simulink model "Ycap_snt"  (R2025b)
settings: Solver=ode45  StartTime=0.0  StopTime=10.0  RelTol=1e-3  EnableMultiTasking=on
undefined symbols (not defined in the file or in its folder): DiscIntNeverNeededParam, Ts
libraries: fl_lib x24, nesl_utility x12
(part 1 of 3)
settings Model: Creator=gdudgeon  LastModifiedBy=gdudgeon
settings SolverCC: AlgebraicLoopSolver=TrustRegion
settings DataIOCC: LimitDataPoints=on  SaveFormat=Array  ReturnWorkspaceOutputs=off
settings OptimizationCC: LifeSpan=inf
settings DebuggingCC: UnderspecifiedInitializationDetection=Classic  MergeDetectMultiDrivingBlocksExec=none  SolverPrmCheckMsg=warning  UnconnectedInputMsg=warning  UnconnectedOutputMsg=warning  UnconnectedLineMsg=warning  StateNameClashWarn=warning  SFUnexpectedBacktrackingDiag=warning  SFNoUnconditionalDefaultTransitionDiag=warning  SFExecutionAtInitializationDiag=none  ArithmeticOperatorsInVariantConditions=warning
settings HardwareCC: ProdBitPerPointer=32.0  ProdBitPerSizeT=32.0  ProdBitPerPtrDiffT=32.0  ProdLargestAtomicFloat=None  ProdIntDivRoundTo=Undefined  ProdEndianess=Unspecified  ProdWordSize=32.0  ProdHWDeviceType=32-bit Generic
settings ModelReferenceCC: EnableRefExpFcnMdlSchedulingChecks=on  PropagateSignalLabelsOutOfModel=off
settings SFSimCC: SimUseLocalCustomCode=off  CustomCodeUndefinedFunction=UseInterfaceOnly
settings RTWCC: RTWUseLocalCustomCode=off  GPUComputeCapability=3.5
settings CodeAppCC: StateflowObjectComments=on
settings GRTTargetCC: TargetLangStandard=C89/C90 (ANSI)
settings ConfigComp: CovMetricSettings=dw  CovSaveCumulativeToWorkspaceVar=on  CovSaveSingleToWorkspaceVar=on  CovExternalEMLEnable=off
settings SimscapeCC: SimscapeNormalizeSystem=off

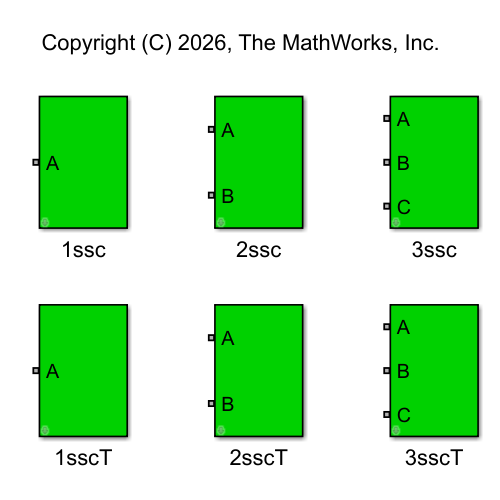
[thumbnail: Simulink's stored preview of the top-level diagram]
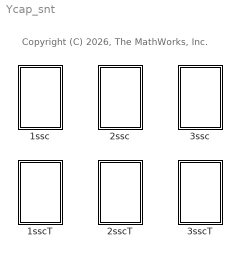
== system Ycap_snt ==
  note: Copyright (C) 2026, The MathWorks, Inc.
  1ssc : Subsystem  mask{V=4.16e3, Qc=50e3}
      mask prompts: V "Vrms (V)"; Qc "Reactive power (VAr)"
  1sscT : Subsystem  mask{V=4.16e3, Qc=50e3}
      mask prompts: V "Vrms (V)"; Qc "Reactive power (VAr)"
  2ssc : Subsystem  mask{V=4.16e3, Qc=50e3}
      mask prompts: V "Vrms (V)"; Qc "Reactive power (VAr)"
  2sscT : Subsystem  mask{V=4.16e3, Qc=50e3}
      mask prompts: V "Vrms (V)"; Qc "Reactive power (VAr)"
  3ssc : Subsystem  mask{V=4.16e3, Qc=200e3}
      mask prompts: V "Vrms (V)"; Qc "Reactive power (VAr)"
  3sscT : Subsystem  mask{V=4.16e3, Qc=200e3}
      mask prompts: V "Vrms (V)"; Qc "Reactive power (VAr)"

== system Ycap_snt/1ssc ==
  Electrical Reference : fl_lib/Electrical/Electrical Elements/Electrical Reference
  cap load : Subsystem  mask{Vrms=V/sqrt(3), f=60, P=0, Q=Qc}
      mask prompts: Vrms "Vrms (V)"; f "freq (Hz)"; P "P (W)"; Q "Q (VA)"
      mask init:
      | R = Vrms^2*P/(P^2 + Q^2);
      | 
      | C = (P^2 + Q^2)/(2*pi*f)/Vrms^2/Q;
  A : PMIOPort  Side=Left
  connections:
  Electrical Reference/LConn1 -- cap load/RConn1
  A/RConn1 -- cap load/LConn1

== system Ycap_snt/1sscT ==
  Constant : Constant  Value=[0 -Qc]  SampleTime=-1
  Electrical Reference1 : fl_lib/Electrical/Electrical Elements/Electrical Reference
  constPQ1 : Subsystem
  A : PMIOPort  Side=Left
  wires:
  Constant/1 -> constPQ1/1(PQ)
  connections:
  constPQ1/RConn1 -- A/RConn1
  constPQ1/LConn1 -- Electrical Reference1/LConn1

== system Ycap_snt/2ssc ==
  Electrical Reference : fl_lib/Electrical/Electrical Elements/Electrical Reference
  cap load : Subsystem  mask{Vrms=V/sqrt(3), f=60, P=0, Q=Qc}
      mask prompts: Vrms "Vrms (V)"; f "freq (Hz)"; P "P (W)"; Q "Q (VA)"
      mask init:
      | R = Vrms^2*P/(P^2 + Q^2);
      | 
      | C = (P^2 + Q^2)/(2*pi*f)/Vrms^2/Q;
  cap load1 : Subsystem  mask{Vrms=V/sqrt(3), f=60, P=0, Q=Qc}
      mask prompts: Vrms "Vrms (V)"; f "freq (Hz)"; P "P (W)"; Q "Q (VA)"
      mask init:
      | R = Vrms^2*P/(P^2 + Q^2);
      | 
      | C = (P^2 + Q^2)/(2*pi*f)/Vrms^2/Q;
  A : PMIOPort  Side=Left
  B : PMIOPort  Port=2  Side=Left
  connections:
  cap load1/LConn1 -- B/RConn1
  cap load/LConn1 -- A/RConn1
  Electrical Reference/LConn1 -- cap load1/RConn1 -- cap load/RConn1

== system Ycap_snt/2sscT ==
  Constant : Constant  Value=[0 -Qc]  SampleTime=-1
  Electrical Reference : fl_lib/Electrical/Electrical Elements/Electrical Reference
  constPQ1 : Subsystem
  constPQ2 : Subsystem
  A : PMIOPort  Side=Left
  B : PMIOPort  Port=2  Side=Left
  wires:
  Constant/1 -> constPQ2/1(PQ), constPQ1/1(PQ)
  connections:
  constPQ1/RConn1 -- A/RConn1
  constPQ2/RConn1 -- B/RConn1
  Electrical Reference/LConn1 -- constPQ2/LConn1 -- constPQ1/LConn1

== system Ycap_snt/3ssc ==
  Electrical Reference : fl_lib/Electrical/Electrical Elements/Electrical Reference
  cap load : Subsystem  mask{Vrms=V/sqrt(3), f=60, P=0, Q=Qc}
      mask prompts: Vrms "Vrms (V)"; f "freq (Hz)"; P "P (W)"; Q "Q (VA)"
      mask init:
      | R = Vrms^2*P/(P^2 + Q^2);
      | 
      | C = (P^2 + Q^2)/(2*pi*f)/Vrms^2/Q;
  cap load1 : Subsystem  mask{Vrms=V/sqrt(3), f=60, P=0, Q=Qc}
      mask prompts: Vrms "Vrms (V)"; f "freq (Hz)"; P "P (W)"; Q "Q (VA)"
      mask init:
      | R = Vrms^2*P/(P^2 + Q^2);
      | 
      | C = (P^2 + Q^2)/(2*pi*f)/Vrms^2/Q;
  cap load2 : Subsystem  mask{Vrms=V/sqrt(3), f=60, P=0, Q=Qc}
      mask prompts: Vrms "Vrms (V)"; f "freq (Hz)"; P "P (W)"; Q "Q (VA)"
      mask init:
      | R = Vrms^2*P/(P^2 + Q^2);
      | 
      | C = (P^2 + Q^2)/(2*pi*f)/Vrms^2/Q;
  A : PMIOPort  Side=Left
  B : PMIOPort  Port=2  Side=Left
  C : PMIOPort  Port=3  Side=Left
  connections:
  cap load2/LConn1 -- C/RConn1
  cap load1/LConn1 -- B/RConn1
  cap load/LConn1 -- A/RConn1
  Electrical Reference/LConn1 -- cap load2/RConn1 -- cap load1/RConn1 -- cap load/RConn1

== system Ycap_snt/3sscT ==
  Constant : Constant  Value=[0 -Qc]  SampleTime=-1
  Electrical Reference : fl_lib/Electrical/Electrical Elements/Electrical Reference
  constPQ1 : Subsystem
  constPQ2 : Subsystem
  constPQ3 : Subsystem
  A : PMIOPort  Side=Left
  B : PMIOPort  Port=2  Side=Left
  C : PMIOPort  Port=3  Side=Left
  wires:
  Constant/1 -> constPQ3/1(PQ), constPQ2/1(PQ), constPQ1/1(PQ)
  connections:
  constPQ1/RConn1 -- A/RConn1
  constPQ2/RConn1 -- B/RConn1
  constPQ3/RConn1 -- C/RConn1
  Electrical Reference/LConn1 -- constPQ3/LConn1 -- constPQ2/LConn1 -- constPQ1/LConn1

== system Ycap_snt/1ssc/cap load ==
  Capacitor : fl_lib/Electrical/Electrical Elements/Capacitor  c=C F  r=R Ohm  g=0 1/Ohm  i_specify=on  i_priority=Low  i=0 A  i_nominal_specify=off  i_nominal_value=1  i_nominal_unit=A  v_specify=on  v_priority=Low  v=0 V  v_nominal_specify=off  v_nominal_value=1  v_nominal_unit=V  vc_specify=on  vc_priority=Low  vc=0 V  vc_nominal_specify=off  vc_nominal_value=1  vc_nominal_unit=V
  " +" : PMIOPort  Side=Left
  - : PMIOPort  Port=2  Side=Right
  connections:
  Capacitor/LConn1 -- " +"/RConn1
  Capacitor/RConn1 -- -/RConn1

== system Ycap_snt/1sscT/constPQ1 ==
  PQ : Inport
  Controlled Current Source : fl_lib/Electrical/Electrical Sources/Controlled Current Source
  Demux : Demux  Outputs=2
  PS-Simulink Converter : nesl_utility/PS-Simulink Converter  PhysicalDomain=network_engine_domain  SubClassName=ps_output  LeftPortType=input  RightPortType=output  PseudoPeriodic=off  Frequencies=[]  VectorFormat=inherit  Unit=inherit  AffineConversion=off
  Simulink-PS Converter : nesl_utility/Simulink-PS Converter  PhysicalDomain=network_engine_domain  SubClassName=ps_input  LeftPortType=input  RightPortType=output  PseudoPeriodic=off  Frequencies=[]  NoiseDistribution=none  NoiseParameters=[]  Unit=1  AffineConversion=off  FilteringAndDerivatives=zero  SimscapeFilterOrder=1  InputFilterTimeConstant=0.001  UdotUserProvided=0
  Voltage Sensor : fl_lib/Electrical/Electrical Sensors/Voltage Sensor
  single-phase PQ : Subsystem
      settings: PortSchema="{\"entries\":[{\"content\":{\"sides\":[{\"content\":{\"connectorIds\":[\"In1\",\"In2\"]},\"type\":\"ConnectorPlacement.EquallySpacedRectSide\",\"uuid\":\"dcb77ad6-d65a-4afe-9b75-44cea2e03bc8\"},{\"content\":{\"connectorIds\":[\"Out1\"],\"side\":\"RIGHT\"},\"type\":\"ConnectorPlacement.EquallySpacedRectSide\",\"uuid\":\"20550ec8-912f-4e6b-8efc-55d7f6680ac4\"},{\"content\":{\"side\":\"TOP\"},\"type\":\"ConnectorPlacement.EquallySpacedRectSide\",\"uuid\":\"6ad8cbf4-1495-4620-97d9-4b8af34d00d1\"},{\"content\":{\"connectorIds\":[\"In3\"],\"side\":\"BOTTOM\"},\"type\":\"ConnectorPlacement.EquallySpacedRectSide\",\"uuid\":\"0b9a8788-8400-4a69-9d07-dd0028530e33\"}]},\"type\":\"ConnectorPlacement.EquallySpacedConnector\",\"uuid\":\"b57ec49b-aa32-43b3-a026-14ed90072d63\"}],\"packageUris\":[\"http://schema.mathworks.com/mf0/Connector/R2020b\"],\"version\":\"1.0\"}"
  + : PMIOPort  Side=Right
  - : PMIOPort  Port=2  Side=Left
  wires:
  PS-Simulink Converter/1 -> single-phase PQ/3(meas)
  single-phase PQ/1(I_1ph) -> Simulink-PS Converter/1
  Demux/1 -> single-phase PQ/1(P)
  Demux/2 -> single-phase PQ/2(Q)
  PQ/1 -> Demux/1
  connections:
  Controlled Current Source/RConn2 -- -/RConn1 -- Voltage Sensor/RConn2
  Voltage Sensor/LConn1 -- +/RConn1 -- Controlled Current Source/LConn1
  PS-Simulink Converter/LConn1 -- Voltage Sensor/RConn1
  Simulink-PS Converter/RConn1 -- Controlled Current Source/RConn1

== system Ycap_snt/2ssc/cap load ==
  Capacitor : fl_lib/Electrical/Electrical Elements/Capacitor  c=C F  r=R Ohm  g=0 1/Ohm  i_specify=on  i_priority=Low  i=0 A  i_nominal_specify=off  i_nominal_value=1  i_nominal_unit=A  v_specify=on  v_priority=Low  v=0 V  v_nominal_specify=off  v_nominal_value=1  v_nominal_unit=V  vc_specify=on  vc_priority=Low  vc=0 V  vc_nominal_specify=off  vc_nominal_value=1  vc_nominal_unit=V
  " +" : PMIOPort  Side=Left
  - : PMIOPort  Port=2  Side=Right
  connections:
  Capacitor/LConn1 -- " +"/RConn1
  Capacitor/RConn1 -- -/RConn1

== system Ycap_snt/2ssc/cap load1 ==
  Capacitor : fl_lib/Electrical/Electrical Elements/Capacitor  c=C F  r=R Ohm  g=0 1/Ohm  i_specify=on  i_priority=Low  i=0 A  i_nominal_specify=off  i_nominal_value=1  i_nominal_unit=A  v_specify=on  v_priority=Low  v=0 V  v_nominal_specify=off  v_nominal_value=1  v_nominal_unit=V  vc_specify=on  vc_priority=Low  vc=0 V  vc_nominal_specify=off  vc_nominal_value=1  vc_nominal_unit=V
  " +" : PMIOPort  Side=Left
  - : PMIOPort  Port=2  Side=Right
  connections:
  Capacitor/RConn1 -- -/RConn1
  Capacitor/LConn1 -- " +"/RConn1

== system Ycap_snt/2sscT/constPQ1 ==
  PQ : Inport
  Controlled Current Source : fl_lib/Electrical/Electrical Sources/Controlled Current Source
  Demux : Demux  Outputs=2
  PS-Simulink Converter : nesl_utility/PS-Simulink Converter  PhysicalDomain=network_engine_domain  SubClassName=ps_output  LeftPortType=input  RightPortType=output  PseudoPeriodic=off  Frequencies=[]  VectorFormat=inherit  Unit=inherit  AffineConversion=off
  Simulink-PS Converter : nesl_utility/Simulink-PS Converter  PhysicalDomain=network_engine_domain  SubClassName=ps_input  LeftPortType=input  RightPortType=output  PseudoPeriodic=off  Frequencies=[]  NoiseDistribution=none  NoiseParameters=[]  Unit=1  AffineConversion=off  FilteringAndDerivatives=zero  SimscapeFilterOrder=1  InputFilterTimeConstant=0.001  UdotUserProvided=0
  Voltage Sensor : fl_lib/Electrical/Electrical Sensors/Voltage Sensor
  single-phase PQ : Subsystem
      settings: PortSchema="{\"entries\":[{\"content\":{\"sides\":[{\"content\":{\"connectorIds\":[\"In1\",\"In2\"]},\"type\":\"ConnectorPlacement.EquallySpacedRectSide\",\"uuid\":\"dcb77ad6-d65a-4afe-9b75-44cea2e03bc8\"},{\"content\":{\"connectorIds\":[\"Out1\"],\"side\":\"RIGHT\"},\"type\":\"ConnectorPlacement.EquallySpacedRectSide\",\"uuid\":\"20550ec8-912f-4e6b-8efc-55d7f6680ac4\"},{\"content\":{\"side\":\"TOP\"},\"type\":\"ConnectorPlacement.EquallySpacedRectSide\",\"uuid\":\"6ad8cbf4-1495-4620-97d9-4b8af34d00d1\"},{\"content\":{\"connectorIds\":[\"In3\"],\"side\":\"BOTTOM\"},\"type\":\"ConnectorPlacement.EquallySpacedRectSide\",\"uuid\":\"0b9a8788-8400-4a69-9d07-dd0028530e33\"}]},\"type\":\"ConnectorPlacement.EquallySpacedConnector\",\"uuid\":\"b57ec49b-aa32-43b3-a026-14ed90072d63\"}],\"packageUris\":[\"http://schema.mathworks.com/mf0/Connector/R2020b\"],\"version\":\"1.0\"}"
  + : PMIOPort  Side=Right
  - : PMIOPort  Port=2  Side=Left
  wires:
  PS-Simulink Converter/1 -> single-phase PQ/3(meas)
  single-phase PQ/1(I_1ph) -> Simulink-PS Converter/1
  Demux/1 -> single-phase PQ/1(P)
  Demux/2 -> single-phase PQ/2(Q)
  PQ/1 -> Demux/1
  connections:
  Controlled Current Source/RConn2 -- -/RConn1 -- Voltage Sensor/RConn2
  Voltage Sensor/LConn1 -- +/RConn1 -- Controlled Current Source/LConn1
  PS-Simulink Converter/LConn1 -- Voltage Sensor/RConn1
  Simulink-PS Converter/RConn1 -- Controlled Current Source/RConn1

== system Ycap_snt/2sscT/constPQ2 ==
  PQ : Inport
  Controlled Current Source : fl_lib/Electrical/Electrical Sources/Controlled Current Source
  Demux : Demux  Outputs=2
  PS-Simulink Converter : nesl_utility/PS-Simulink Converter  PhysicalDomain=network_engine_domain  SubClassName=ps_output  LeftPortType=input  RightPortType=output  PseudoPeriodic=off  Frequencies=[]  VectorFormat=inherit  Unit=inherit  AffineConversion=off
  Simulink-PS Converter : nesl_utility/Simulink-PS Converter  PhysicalDomain=network_engine_domain  SubClassName=ps_input  LeftPortType=input  RightPortType=output  PseudoPeriodic=off  Frequencies=[]  NoiseDistribution=none  NoiseParameters=[]  Unit=1  AffineConversion=off  FilteringAndDerivatives=zero  SimscapeFilterOrder=1  InputFilterTimeConstant=0.001  UdotUserProvided=0
  Voltage Sensor : fl_lib/Electrical/Electrical Sensors/Voltage Sensor
  single-phase PQ : Subsystem
      settings: PortSchema="{\"entries\":[{\"content\":{\"sides\":[{\"content\":{\"connectorIds\":[\"In1\",\"In2\"]},\"type\":\"ConnectorPlacement.EquallySpacedRectSide\",\"uuid\":\"dcb77ad6-d65a-4afe-9b75-44cea2e03bc8\"},{\"content\":{\"connectorIds\":[\"Out1\"],\"side\":\"RIGHT\"},\"type\":\"ConnectorPlacement.EquallySpacedRectSide\",\"uuid\":\"20550ec8-912f-4e6b-8efc-55d7f6680ac4\"},{\"content\":{\"side\":\"TOP\"},\"type\":\"ConnectorPlacement.EquallySpacedRectSide\",\"uuid\":\"6ad8cbf4-1495-4620-97d9-4b8af34d00d1\"},{\"content\":{\"connectorIds\":[\"In3\"],\"side\":\"BOTTOM\"},\"type\":\"ConnectorPlacement.EquallySpacedRectSide\",\"uuid\":\"0b9a8788-8400-4a69-9d07-dd0028530e33\"}]},\"type\":\"ConnectorPlacement.EquallySpacedConnector\",\"uuid\":\"b57ec49b-aa32-43b3-a026-14ed90072d63\"}],\"packageUris\":[\"http://schema.mathworks.com/mf0/Connector/R2020b\"],\"version\":\"1.0\"}"
  + : PMIOPort  Side=Right
  - : PMIOPort  Port=2  Side=Left
  wires:
  PQ/1 -> Demux/1
  Demux/2 -> single-phase PQ/2(Q)
  Demux/1 -> single-phase PQ/1(P)
  single-phase PQ/1(I_1ph) -> Simulink-PS Converter/1
  PS-Simulink Converter/1 -> single-phase PQ/3(meas)
  connections:
  Simulink-PS Converter/RConn1 -- Controlled Current Source/RConn1
  PS-Simulink Converter/LConn1 -- Voltage Sensor/RConn1
  Controlled Current Source/LConn1 -- +/RConn1 -- Voltage Sensor/LConn1
  Voltage Sensor/RConn2 -- -/RConn1 -- Controlled Current Source/RConn2

== system Ycap_snt/3ssc/cap load ==
  Capacitor : fl_lib/Electrical/Electrical Elements/Capacitor  c=C F  r=R Ohm  g=0 1/Ohm  i_specify=on  i_priority=Low  i=0 A  i_nominal_specify=off  i_nominal_value=1  i_nominal_unit=A  v_specify=on  v_priority=Low  v=0 V  v_nominal_specify=off  v_nominal_value=1  v_nominal_unit=V  vc_specify=on  vc_priority=Low  vc=0 V  vc_nominal_specify=off  vc_nominal_value=1  vc_nominal_unit=V
  " +" : PMIOPort  Side=Left
  - : PMIOPort  Port=2  Side=Right
  connections:
  Capacitor/LConn1 -- " +"/RConn1
  Capacitor/RConn1 -- -/RConn1

== system Ycap_snt/3ssc/cap load1 ==
  Capacitor : fl_lib/Electrical/Electrical Elements/Capacitor  c=C F  r=R Ohm  g=0 1/Ohm  i_specify=on  i_priority=Low  i=0 A  i_nominal_specify=off  i_nominal_value=1  i_nominal_unit=A  v_specify=on  v_priority=Low  v=0 V  v_nominal_specify=off  v_nominal_value=1  v_nominal_unit=V  vc_specify=on  vc_priority=Low  vc=0 V  vc_nominal_specify=off  vc_nominal_value=1  vc_nominal_unit=V
  " +" : PMIOPort  Side=Left
  - : PMIOPort  Port=2  Side=Right
  connections:
  Capacitor/RConn1 -- -/RConn1
  Capacitor/LConn1 -- " +"/RConn1

== system Ycap_snt/3ssc/cap load2 ==
  Capacitor : fl_lib/Electrical/Electrical Elements/Capacitor  c=C F  r=R Ohm  g=0 1/Ohm  i_specify=on  i_priority=Low  i=0 A  i_nominal_specify=off  i_nominal_value=1  i_nominal_unit=A  v_specify=on  v_priority=Low  v=0 V  v_nominal_specify=off  v_nominal_value=1  v_nominal_unit=V  vc_specify=on  vc_priority=Low  vc=0 V  vc_nominal_specify=off  vc_nominal_value=1  vc_nominal_unit=V
  " +" : PMIOPort  Side=Left
  - : PMIOPort  Port=2  Side=Right
  connections:
  Capacitor/LConn1 -- " +"/RConn1
  Capacitor/RConn1 -- -/RConn1

== system Ycap_snt/3sscT/constPQ1 ==
  PQ : Inport
  Controlled Current Source : fl_lib/Electrical/Electrical Sources/Controlled Current Source
  Demux : Demux  Outputs=2
  PS-Simulink Converter : nesl_utility/PS-Simulink Converter  PhysicalDomain=network_engine_domain  SubClassName=ps_output  LeftPortType=input  RightPortType=output  PseudoPeriodic=off  Frequencies=[]  VectorFormat=inherit  Unit=inherit  AffineConversion=off
  Simulink-PS Converter : nesl_utility/Simulink-PS Converter  PhysicalDomain=network_engine_domain  SubClassName=ps_input  LeftPortType=input  RightPortType=output  PseudoPeriodic=off  Frequencies=[]  NoiseDistribution=none  NoiseParameters=[]  Unit=1  AffineConversion=off  FilteringAndDerivatives=zero  SimscapeFilterOrder=1  InputFilterTimeConstant=0.001  UdotUserProvided=0
  Voltage Sensor : fl_lib/Electrical/Electrical Sensors/Voltage Sensor
  single-phase PQ : Subsystem
      settings: PortSchema="{\"entries\":[{\"content\":{\"sides\":[{\"content\":{\"connectorIds\":[\"In1\",\"In2\"]},\"type\":\"ConnectorPlacement.EquallySpacedRectSide\",\"uuid\":\"dcb77ad6-d65a-4afe-9b75-44cea2e03bc8\"},{\"content\":{\"connectorIds\":[\"Out1\"],\"side\":\"RIGHT\"},\"type\":\"ConnectorPlacement.EquallySpacedRectSide\",\"uuid\":\"20550ec8-912f-4e6b-8efc-55d7f6680ac4\"},{\"content\":{\"side\":\"TOP\"},\"type\":\"ConnectorPlacement.EquallySpacedRectSide\",\"uuid\":\"6ad8cbf4-1495-4620-97d9-4b8af34d00d1\"},{\"content\":{\"connectorIds\":[\"In3\"],\"side\":\"BOTTOM\"},\"type\":\"ConnectorPlacement.EquallySpacedRectSide\",\"uuid\":\"0b9a8788-8400-4a69-9d07-dd0028530e33\"}]},\"type\":\"ConnectorPlacement.EquallySpacedConnector\",\"uuid\":\"b57ec49b-aa32-43b3-a026-14ed90072d63\"}],\"packageUris\":[\"http://schema.mathworks.com/mf0/Connector/R2020b\"],\"version\":\"1.0\"}"
  + : PMIOPort  Side=Right
  - : PMIOPort  Port=2  Side=Left
  wires:
  PS-Simulink Converter/1 -> single-phase PQ/3(meas)
  single-phase PQ/1(I_1ph) -> Simulink-PS Converter/1
  Demux/1 -> single-phase PQ/1(P)
  Demux/2 -> single-phase PQ/2(Q)
  PQ/1 -> Demux/1
  connections:
  Controlled Current Source/RConn2 -- -/RConn1 -- Voltage Sensor/RConn2
  Voltage Sensor/LConn1 -- +/RConn1 -- Controlled Current Source/LConn1
  PS-Simulink Converter/LConn1 -- Voltage Sensor/RConn1
  Simulink-PS Converter/RConn1 -- Controlled Current Source/RConn1

== system Ycap_snt/3sscT/constPQ2 ==
  PQ : Inport
  Controlled Current Source : fl_lib/Electrical/Electrical Sources/Controlled Current Source
  Demux : Demux  Outputs=2
  PS-Simulink Converter : nesl_utility/PS-Simulink Converter  PhysicalDomain=network_engine_domain  SubClassName=ps_output  LeftPortType=input  RightPortType=output  PseudoPeriodic=off  Frequencies=[]  VectorFormat=inherit  Unit=inherit  AffineConversion=off
  Simulink-PS Converter : nesl_utility/Simulink-PS Converter  PhysicalDomain=network_engine_domain  SubClassName=ps_input  LeftPortType=input  RightPortType=output  PseudoPeriodic=off  Frequencies=[]  NoiseDistribution=none  NoiseParameters=[]  Unit=1  AffineConversion=off  FilteringAndDerivatives=zero  SimscapeFilterOrder=1  InputFilterTimeConstant=0.001  UdotUserProvided=0
  Voltage Sensor : fl_lib/Electrical/Electrical Sensors/Voltage Sensor
  single-phase PQ : Subsystem
      settings: PortSchema="{\"entries\":[{\"content\":{\"sides\":[{\"content\":{\"connectorIds\":[\"In1\",\"In2\"]},\"type\":\"ConnectorPlacement.EquallySpacedRectSide\",\"uuid\":\"dcb77ad6-d65a-4afe-9b75-44cea2e03bc8\"},{\"content\":{\"connectorIds\":[\"Out1\"],\"side\":\"RIGHT\"},\"type\":\"ConnectorPlacement.EquallySpacedRectSide\",\"uuid\":\"20550ec8-912f-4e6b-8efc-55d7f6680ac4\"},{\"content\":{\"side\":\"TOP\"},\"type\":\"ConnectorPlacement.EquallySpacedRectSide\",\"uuid\":\"6ad8cbf4-1495-4620-97d9-4b8af34d00d1\"},{\"content\":{\"connectorIds\":[\"In3\"],\"side\":\"BOTTOM\"},\"type\":\"ConnectorPlacement.EquallySpacedRectSide\",\"uuid\":\"0b9a8788-8400-4a69-9d07-dd0028530e33\"}]},\"type\":\"ConnectorPlacement.EquallySpacedConnector\",\"uuid\":\"b57ec49b-aa32-43b3-a026-14ed90072d63\"}],\"packageUris\":[\"http://schema.mathworks.com/mf0/Connector/R2020b\"],\"version\":\"1.0\"}"
  + : PMIOPort  Side=Right
  - : PMIOPort  Port=2  Side=Left
  wires:
  PQ/1 -> Demux/1
  Demux/2 -> single-phase PQ/2(Q)
  Demux/1 -> single-phase PQ/1(P)
  single-phase PQ/1(I_1ph) -> Simulink-PS Converter/1
  PS-Simulink Converter/1 -> single-phase PQ/3(meas)
  connections:
  Simulink-PS Converter/RConn1 -- Controlled Current Source/RConn1
  PS-Simulink Converter/LConn1 -- Voltage Sensor/RConn1
  Controlled Current Source/LConn1 -- +/RConn1 -- Voltage Sensor/LConn1
  Voltage Sensor/RConn2 -- -/RConn1 -- Controlled Current Source/RConn2

== system Ycap_snt/3sscT/constPQ3 ==
  PQ : Inport
  Controlled Current Source : fl_lib/Electrical/Electrical Sources/Controlled Current Source
  Demux : Demux  Outputs=2
  PS-Simulink Converter : nesl_utility/PS-Simulink Converter  PhysicalDomain=network_engine_domain  SubClassName=ps_output  LeftPortType=input  RightPortType=output  PseudoPeriodic=off  Frequencies=[]  VectorFormat=inherit  Unit=inherit  AffineConversion=off
  Simulink-PS Converter : nesl_utility/Simulink-PS Converter  PhysicalDomain=network_engine_domain  SubClassName=ps_input  LeftPortType=input  RightPortType=output  PseudoPeriodic=off  Frequencies=[]  NoiseDistribution=none  NoiseParameters=[]  Unit=1  AffineConversion=off  FilteringAndDerivatives=zero  SimscapeFilterOrder=1  InputFilterTimeConstant=0.001  UdotUserProvided=0
  Voltage Sensor : fl_lib/Electrical/Electrical Sensors/Voltage Sensor
  single-phase PQ : Subsystem
      settings: PortSchema="{\"entries\":[{\"content\":{\"sides\":[{\"content\":{\"connectorIds\":[\"In1\",\"In2\"]},\"type\":\"ConnectorPlacement.EquallySpacedRectSide\",\"uuid\":\"dcb77ad6-d65a-4afe-9b75-44cea2e03bc8\"},{\"content\":{\"connectorIds\":[\"Out1\"],\"side\":\"RIGHT\"},\"type\":\"ConnectorPlacement.EquallySpacedRectSide\",\"uuid\":\"20550ec8-912f-4e6b-8efc-55d7f6680ac4\"},{\"content\":{\"side\":\"TOP\"},\"type\":\"ConnectorPlacement.EquallySpacedRectSide\",\"uuid\":\"6ad8cbf4-1495-4620-97d9-4b8af34d00d1\"},{\"content\":{\"connectorIds\":[\"In3\"],\"side\":\"BOTTOM\"},\"type\":\"ConnectorPlacement.EquallySpacedRectSide\",\"uuid\":\"0b9a8788-8400-4a69-9d07-dd0028530e33\"}]},\"type\":\"ConnectorPlacement.EquallySpacedConnector\",\"uuid\":\"b57ec49b-aa32-43b3-a026-14ed90072d63\"}],\"packageUris\":[\"http://schema.mathworks.com/mf0/Connector/R2020b\"],\"version\":\"1.0\"}"
  + : PMIOPort  Side=Right
  - : PMIOPort  Port=2  Side=Left
  wires:
  PS-Simulink Converter/1 -> single-phase PQ/3(meas)
  single-phase PQ/1(I_1ph) -> Simulink-PS Converter/1
  Demux/1 -> single-phase PQ/1(P)
  Demux/2 -> single-phase PQ/2(Q)
  PQ/1 -> Demux/1
  connections:
  Controlled Current Source/RConn2 -- -/RConn1 -- Voltage Sensor/RConn2
  Voltage Sensor/LConn1 -- +/RConn1 -- Controlled Current Source/LConn1
  PS-Simulink Converter/LConn1 -- Voltage Sensor/RConn1
  Simulink-PS Converter/RConn1 -- Controlled Current Source/RConn1

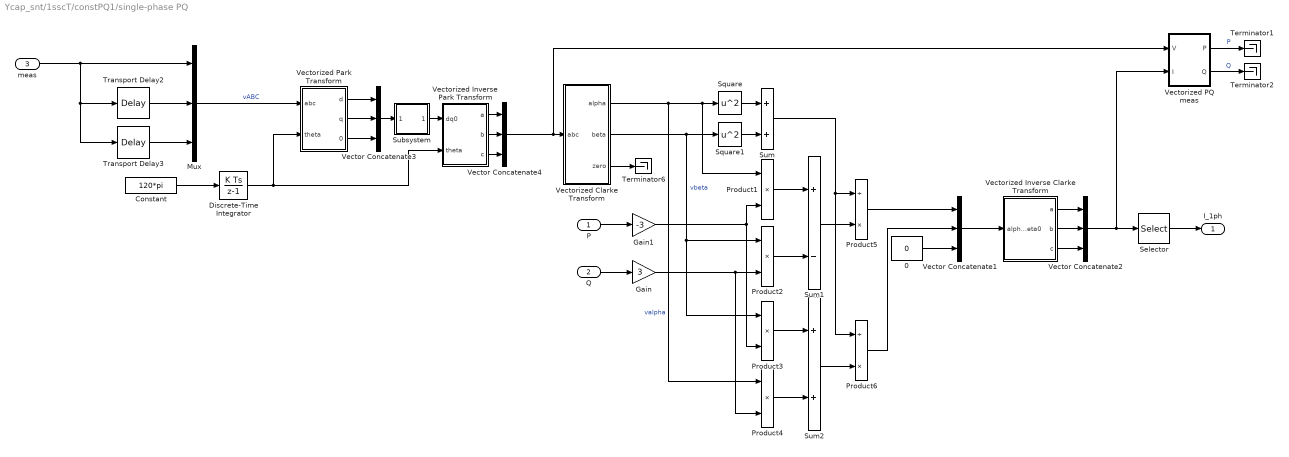
== system Ycap_snt/1sscT/constPQ1/single-phase PQ ==
  P : Inport
  Q : Inport  Port=2
  meas : Inport  Port=3
  "0 " : Constant  Value=0  VectorParams1D=off  SampleTime=Ts
  Constant : Constant  Value=120*pi  VectorParams1D=off  SampleTime=Ts
  Discrete-Time Integrator : DiscreteIntegrator  SampleTime=Ts  ICPrevOutput=DiscIntNeverNeededParam  ICPrevScaledInput=DiscIntNeverNeededParam
  Gain : Gain  Gain=3
  Gain1 : Gain  Gain=-3
  Mux : Mux  Inputs=3
  Product{1..4} (4 alike) : Product
  Product5 : Product  Inputs=/*
  Product6 : Product  Inputs=/*
  Selector : Selector  InputPortWidth=3  IndexOptions=Index vector (dialog)  Indices=1  OutputSizes=1
  Square : Math  Operator=square
  Square1 : Math  Operator=square
  Subsystem : Subsystem
  Sum : Sum
  Sum1 : Sum  Inputs=+-
  Sum2 : Sum
  Terminator1 : Terminator
  Terminator2 : Terminator
  Terminator6 : Terminator
  Transport Delay2 : TransportDelay  DelayTime=1/180
  Transport Delay3 : TransportDelay  DelayTime=2/180
  Vector Concatenate{1..4} (4 alike) : Concatenate  NumInputs=3  Mode=Multidimensional array
  Vectorized Clarke Transform : Subsystem  mask{no_meas=1}
      mask prompts: no_meas "Number of measurements"
  Vectorized PQ meas : Subsystem  DialogController=POWERSYS.PowerSysDialog
  Vectorized Park Transform : Subsystem  mask{no_meas=1}
      mask prompts: no_meas "Number of measurements"
  Vectorized Inverse Clarke Transform : Subsystem  mask{no_meas=1}
      mask prompts: no_meas "Number of Measurements"
      mask Display:
      | port_label('input', 1, '\alpha\beta0', 'texmode', 'on')
      | port_label('output',1,'a')
      | port_label('output',2,'b')
      | port_label('output',3,'c')
  Vectorized Inverse Park Transform : Subsystem  mask{no_meas=1}
      mask prompts: no_meas "Number of Measurements"
  I_1ph : Outport
  wires:
  Sum2/1 -> Product6/2
  Sum/1 -> Product5/1, Product6/1
  P/1 -> Gain1/1
  Square1/1 -> Sum/2
  Product3/1 -> Sum2/1
  Vectorized Clarke Transform/2(beta) -> Product3/1, Product2/1, Square1/1  "vbeta"
  Q/1 -> Gain/1
  "0 "/1 -> Vector Concatenate1/3
  Sum1/1 -> Product5/2
  Vectorized Inverse Clarke Transform/1(a) -> Vector Concatenate2/1
  Vectorized Inverse Clarke Transform/2(b) -> Vector Concatenate2/2
  Vectorized Clarke Transform/3(zero) -> Terminator6/1
  Product2/1 -> Sum1/2
  Vectorized Clarke Transform/1(alpha) -> Product4/1, Product1/1, Square/1  "valpha"
  Product6/1 -> Vector Concatenate1/2
  Product4/1 -> Sum2/2
  Vectorized Inverse Clarke Transform/3(c) -> Vector Concatenate2/3
  Product1/1 -> Sum1/1
  Vector Concatenate1/1 -> Vectorized Inverse Clarke Transform/1(alphabeta0)
  Square/1 -> Sum/1
  Product5/1 -> Vector Concatenate1/1
  Vectorized PQ meas/1(P) -> Terminator1/1  "P"
  Vectorized PQ meas/2(Q) -> Terminator2/1  "Q"
  Vector Concatenate2/1 -> Selector/1, Vectorized PQ meas/2(I)
  Vectorized Park Transform/1(d) -> Vector Concatenate3/1
  Vectorized Park Transform/2(q) -> Vector Concatenate3/2
  Vectorized Park Transform/3(0) -> Vector Concatenate3/3
  Vectorized Inverse Park Transform/1(a) -> Vector Concatenate4/1
  Vectorized Inverse Park Transform/2(b) -> Vector Concatenate4/2
  Vectorized Inverse Park Transform/3(c) -> Vector Concatenate4/3
  Vector Concatenate4/1 -> Vectorized Clarke Transform/1(abc), Vectorized PQ meas/1(V)
  Constant/1 -> Discrete-Time Integrator/1
  Discrete-Time Integrator/1 -> Vectorized Inverse Park Transform/2(theta), Vectorized Park Transform/2(theta)
  Vector Concatenate3/1 -> Subsystem/1(In1)
  Subsystem/1(Out1) -> Vectorized Inverse Park Transform/1(dq0)
  Transport Delay3/1 -> Mux/3
  meas/1 -> Transport Delay3/1, Transport Delay2/1, Mux/1
  Transport Delay2/1 -> Mux/2
  Gain/1 -> Product4/2, Product2/2
  Gain1/1 -> Product1/2, Product3/2
  Mux/1 -> Vectorized Park Transform/1(abc)  "vABC"
  Selector/1 -> I_1ph/1

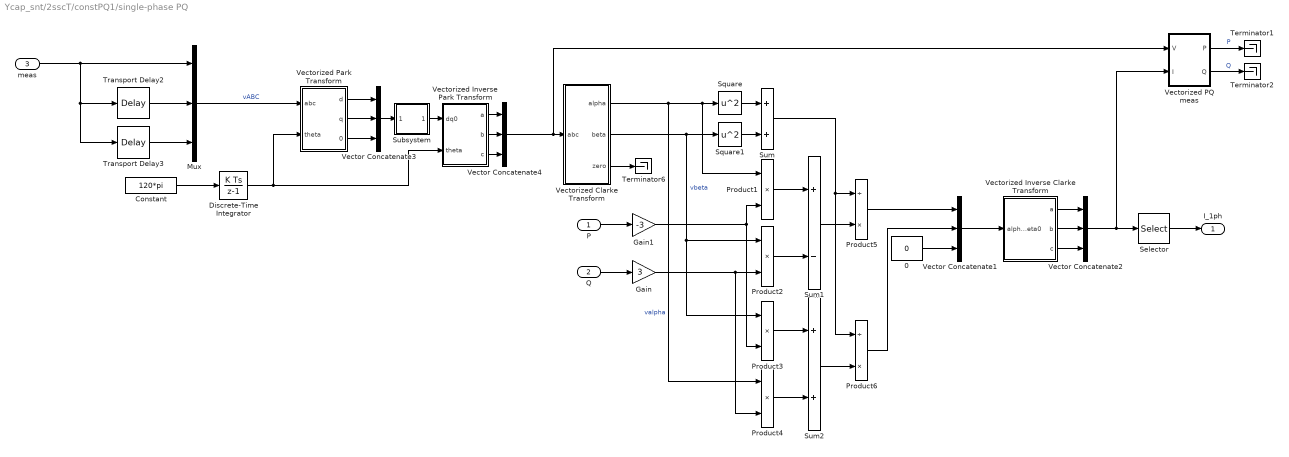
== system Ycap_snt/2sscT/constPQ1/single-phase PQ ==
  P : Inport
  Q : Inport  Port=2
  meas : Inport  Port=3
  "0 " : Constant  Value=0  VectorParams1D=off  SampleTime=Ts
  Constant : Constant  Value=120*pi  VectorParams1D=off  SampleTime=Ts
  Discrete-Time Integrator : DiscreteIntegrator  SampleTime=Ts  ICPrevOutput=DiscIntNeverNeededParam  ICPrevScaledInput=DiscIntNeverNeededParam
  Gain : Gain  Gain=3
  Gain1 : Gain  Gain=-3
  Mux : Mux  Inputs=3
  Product{1..4} (4 alike) : Product
  Product5 : Product  Inputs=/*
  Product6 : Product  Inputs=/*
  Selector : Selector  InputPortWidth=3  IndexOptions=Index vector (dialog)  Indices=1  OutputSizes=1
  Square : Math  Operator=square
  Square1 : Math  Operator=square
  Subsystem : Subsystem
  Sum : Sum
  Sum1 : Sum  Inputs=+-
  Sum2 : Sum
  Terminator1 : Terminator
  Terminator2 : Terminator
  Terminator6 : Terminator
  Transport Delay2 : TransportDelay  DelayTime=1/180
  Transport Delay3 : TransportDelay  DelayTime=2/180
  Vector Concatenate{1..4} (4 alike) : Concatenate  NumInputs=3  Mode=Multidimensional array
  Vectorized Clarke Transform : Subsystem  mask{no_meas=1}
      mask prompts: no_meas "Number of measurements"
  Vectorized PQ meas : Subsystem  DialogController=POWERSYS.PowerSysDialog
  Vectorized Park Transform : Subsystem  mask{no_meas=1}
      mask prompts: no_meas "Number of measurements"
  Vectorized Inverse Clarke Transform : Subsystem  mask{no_meas=1}
      mask prompts: no_meas "Number of Measurements"
      mask Display:
      | port_label('input', 1, '\alpha\beta0', 'texmode', 'on')
      | port_label('output',1,'a')
      | port_label('output',2,'b')
      | port_label('output',3,'c')
  Vectorized Inverse Park Transform : Subsystem  mask{no_meas=1}
      mask prompts: no_meas "Number of Measurements"
  I_1ph : Outport
  wires:
  Sum2/1 -> Product6/2
  Sum/1 -> Product5/1, Product6/1
  P/1 -> Gain1/1
  Square1/1 -> Sum/2
  Product3/1 -> Sum2/1
  Vectorized Clarke Transform/2(beta) -> Product3/1, Product2/1, Square1/1  "vbeta"
  Q/1 -> Gain/1
  "0 "/1 -> Vector Concatenate1/3
  Sum1/1 -> Product5/2
  Vectorized Inverse Clarke Transform/1(a) -> Vector Concatenate2/1
  Vectorized Inverse Clarke Transform/2(b) -> Vector Concatenate2/2
  Vectorized Clarke Transform/3(zero) -> Terminator6/1
  Product2/1 -> Sum1/2
  Vectorized Clarke Transform/1(alpha) -> Product4/1, Product1/1, Square/1  "valpha"
  Product6/1 -> Vector Concatenate1/2
  Product4/1 -> Sum2/2
  Vectorized Inverse Clarke Transform/3(c) -> Vector Concatenate2/3
  Product1/1 -> Sum1/1
  Vector Concatenate1/1 -> Vectorized Inverse Clarke Transform/1(alphabeta0)
  Square/1 -> Sum/1
  Product5/1 -> Vector Concatenate1/1
  Vectorized PQ meas/1(P) -> Terminator1/1  "P"
  Vectorized PQ meas/2(Q) -> Terminator2/1  "Q"
  Vector Concatenate2/1 -> Selector/1, Vectorized PQ meas/2(I)
  Vectorized Park Transform/1(d) -> Vector Concatenate3/1
  Vectorized Park Transform/2(q) -> Vector Concatenate3/2
  Vectorized Park Transform/3(0) -> Vector Concatenate3/3
  Vectorized Inverse Park Transform/1(a) -> Vector Concatenate4/1
  Vectorized Inverse Park Transform/2(b) -> Vector Concatenate4/2
  Vectorized Inverse Park Transform/3(c) -> Vector Concatenate4/3
  Vector Concatenate4/1 -> Vectorized Clarke Transform/1(abc), Vectorized PQ meas/1(V)
  Constant/1 -> Discrete-Time Integrator/1
  Discrete-Time Integrator/1 -> Vectorized Inverse Park Transform/2(theta), Vectorized Park Transform/2(theta)
  Vector Concatenate3/1 -> Subsystem/1(In1)
  Subsystem/1(Out1) -> Vectorized Inverse Park Transform/1(dq0)
  Transport Delay3/1 -> Mux/3
  meas/1 -> Transport Delay3/1, Transport Delay2/1, Mux/1
  Transport Delay2/1 -> Mux/2
  Gain/1 -> Product4/2, Product2/2
  Gain1/1 -> Product1/2, Product3/2
  Mux/1 -> Vectorized Park Transform/1(abc)  "vABC"
  Selector/1 -> I_1ph/1

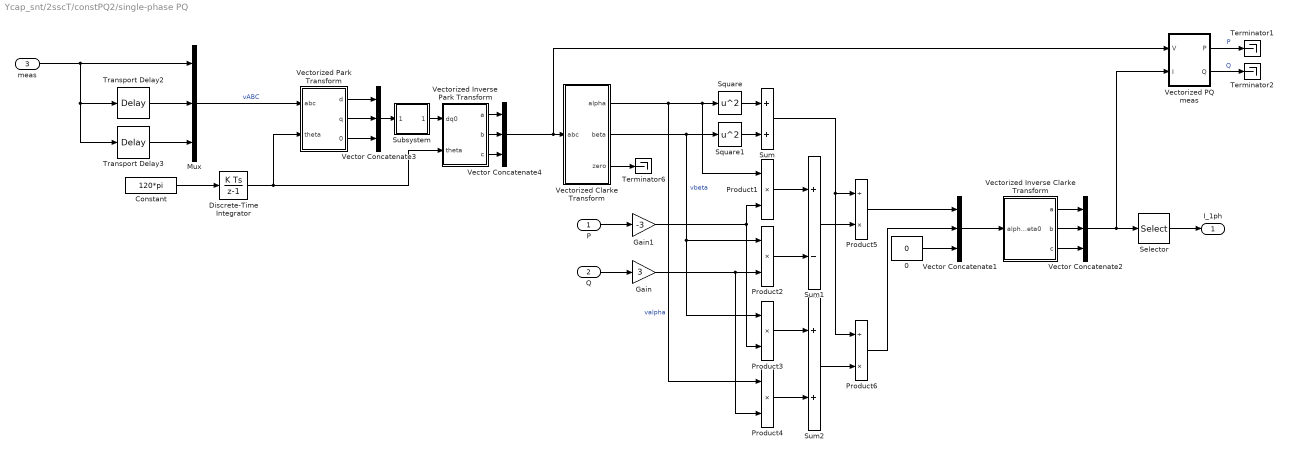
== system Ycap_snt/2sscT/constPQ2/single-phase PQ ==
  P : Inport
  Q : Inport  Port=2
  meas : Inport  Port=3
  "0 " : Constant  Value=0  VectorParams1D=off  SampleTime=Ts
  Constant : Constant  Value=120*pi  VectorParams1D=off  SampleTime=Ts
  Discrete-Time Integrator : DiscreteIntegrator  SampleTime=Ts  ICPrevOutput=DiscIntNeverNeededParam  ICPrevScaledInput=DiscIntNeverNeededParam
  Gain : Gain  Gain=3
  Gain1 : Gain  Gain=-3
  Mux : Mux  Inputs=3
  Product{1..4} (4 alike) : Product
  Product5 : Product  Inputs=/*
  Product6 : Product  Inputs=/*
  Selector : Selector  InputPortWidth=3  IndexOptions=Index vector (dialog)  Indices=1  OutputSizes=1
  Square : Math  Operator=square
  Square1 : Math  Operator=square
  Subsystem : Subsystem
  Sum : Sum
  Sum1 : Sum  Inputs=+-
  Sum2 : Sum
  Terminator1 : Terminator
  Terminator2 : Terminator
  Terminator6 : Terminator
  Transport Delay2 : TransportDelay  DelayTime=1/180
  Transport Delay3 : TransportDelay  DelayTime=2/180
  Vector Concatenate{1..4} (4 alike) : Concatenate  NumInputs=3  Mode=Multidimensional array
  Vectorized Clarke Transform : Subsystem  mask{no_meas=1}
      mask prompts: no_meas "Number of measurements"
  Vectorized PQ meas : Subsystem  DialogController=POWERSYS.PowerSysDialog
  Vectorized Park Transform : Subsystem  mask{no_meas=1}
      mask prompts: no_meas "Number of measurements"
  Vectorized Inverse Clarke Transform : Subsystem  mask{no_meas=1}
      mask prompts: no_meas "Number of Measurements"
      mask Display:
      | port_label('input', 1, '\alpha\beta0', 'texmode', 'on')
      | port_label('output',1,'a')
      | port_label('output',2,'b')
      | port_label('output',3,'c')
  Vectorized Inverse Park Transform : Subsystem  mask{no_meas=1}
      mask prompts: no_meas "Number of Measurements"
  I_1ph : Outport
  wires:
  Selector/1 -> I_1ph/1
  Mux/1 -> Vectorized Park Transform/1(abc)  "vABC"
  Gain1/1 -> Product3/2, Product1/2
  Gain/1 -> Product2/2, Product4/2
  Transport Delay2/1 -> Mux/2
  meas/1 -> Mux/1, Transport Delay2/1, Transport Delay3/1
  Transport Delay3/1 -> Mux/3
  Subsystem/1(Out1) -> Vectorized Inverse Park Transform/1(dq0)
  Vector Concatenate3/1 -> Subsystem/1(In1)
  Discrete-Time Integrator/1 -> Vectorized Park Transform/2(theta), Vectorized Inverse Park Transform/2(theta)
  Constant/1 -> Discrete-Time Integrator/1
  Vector Concatenate4/1 -> Vectorized PQ meas/1(V), Vectorized Clarke Transform/1(abc)
  Vectorized Inverse Park Transform/3(c) -> Vector Concatenate4/3
  Vectorized Inverse Park Transform/2(b) -> Vector Concatenate4/2
  Vectorized Inverse Park Transform/1(a) -> Vector Concatenate4/1
  Vectorized Park Transform/3(0) -> Vector Concatenate3/3
  Vectorized Park Transform/2(q) -> Vector Concatenate3/2
  Vectorized Park Transform/1(d) -> Vector Concatenate3/1
  Vector Concatenate2/1 -> Vectorized PQ meas/2(I), Selector/1
  Vectorized PQ meas/2(Q) -> Terminator2/1  "Q"
  Vectorized PQ meas/1(P) -> Terminator1/1  "P"
  Product5/1 -> Vector Concatenate1/1
  Square/1 -> Sum/1
  Vector Concatenate1/1 -> Vectorized Inverse Clarke Transform/1(alphabeta0)
  Product1/1 -> Sum1/1
  Vectorized Inverse Clarke Transform/3(c) -> Vector Concatenate2/3
  Product4/1 -> Sum2/2
  Product6/1 -> Vector Concatenate1/2
  Vectorized Clarke Transform/1(alpha) -> Square/1, Product1/1, Product4/1  "valpha"
  Product2/1 -> Sum1/2
  Vectorized Clarke Transform/3(zero) -> Terminator6/1
  Vectorized Inverse Clarke Transform/2(b) -> Vector Concatenate2/2
  Vectorized Inverse Clarke Transform/1(a) -> Vector Concatenate2/1
  Sum1/1 -> Product5/2
  "0 "/1 -> Vector Concatenate1/3
  Q/1 -> Gain/1
  Vectorized Clarke Transform/2(beta) -> Square1/1, Product2/1, Product3/1  "vbeta"
  Product3/1 -> Sum2/1
  Square1/1 -> Sum/2
  P/1 -> Gain1/1
  Sum/1 -> Product6/1, Product5/1
  Sum2/1 -> Product6/2

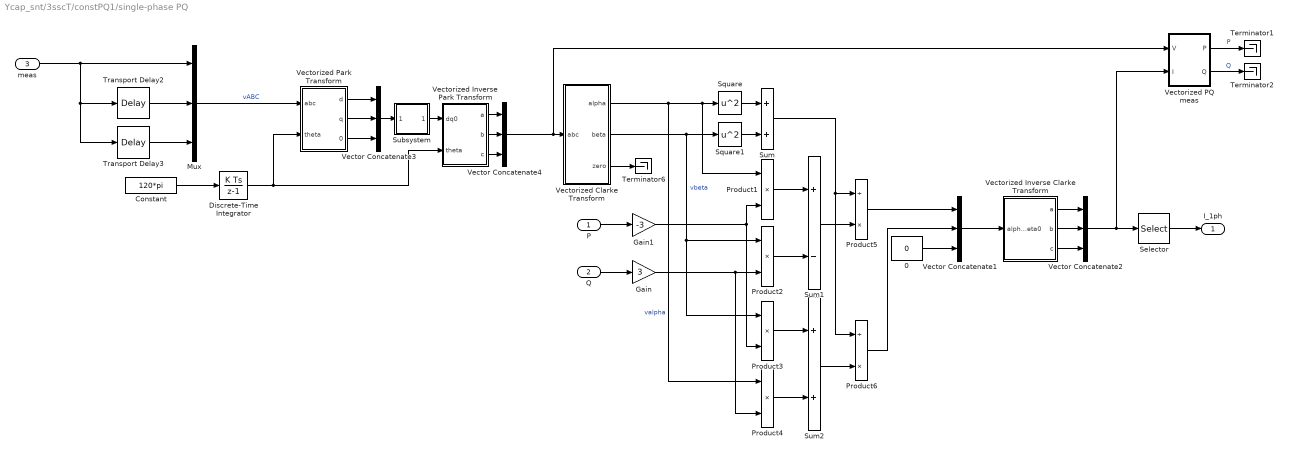
== system Ycap_snt/3sscT/constPQ1/single-phase PQ ==
  P : Inport
  Q : Inport  Port=2
  meas : Inport  Port=3
  "0 " : Constant  Value=0  VectorParams1D=off  SampleTime=Ts
  Constant : Constant  Value=120*pi  VectorParams1D=off  SampleTime=Ts
  Discrete-Time Integrator : DiscreteIntegrator  SampleTime=Ts  ICPrevOutput=DiscIntNeverNeededParam  ICPrevScaledInput=DiscIntNeverNeededParam
  Gain : Gain  Gain=3
  Gain1 : Gain  Gain=-3
  Mux : Mux  Inputs=3
  Product{1..4} (4 alike) : Product
  Product5 : Product  Inputs=/*
  Product6 : Product  Inputs=/*
  Selector : Selector  InputPortWidth=3  IndexOptions=Index vector (dialog)  Indices=1  OutputSizes=1
  Square : Math  Operator=square
  Square1 : Math  Operator=square
  Subsystem : Subsystem
  Sum : Sum
  Sum1 : Sum  Inputs=+-
  Sum2 : Sum
  Terminator1 : Terminator
  Terminator2 : Terminator
  Terminator6 : Terminator
  Transport Delay2 : TransportDelay  DelayTime=1/180
  Transport Delay3 : TransportDelay  DelayTime=2/180
  Vector Concatenate{1..4} (4 alike) : Concatenate  NumInputs=3  Mode=Multidimensional array
  Vectorized Clarke Transform : Subsystem  mask{no_meas=1}
      mask prompts: no_meas "Number of measurements"
  Vectorized PQ meas : Subsystem  DialogController=POWERSYS.PowerSysDialog
  Vectorized Park Transform : Subsystem  mask{no_meas=1}
      mask prompts: no_meas "Number of measurements"
  Vectorized Inverse Clarke Transform : Subsystem  mask{no_meas=1}
      mask prompts: no_meas "Number of Measurements"
      mask Display:
      | port_label('input', 1, '\alpha\beta0', 'texmode', 'on')
      | port_label('output',1,'a')
      | port_label('output',2,'b')
      | port_label('output',3,'c')
  Vectorized Inverse Park Transform : Subsystem  mask{no_meas=1}
      mask prompts: no_meas "Number of Measurements"
  I_1ph : Outport
  wires:
  Sum2/1 -> Product6/2
  Sum/1 -> Product5/1, Product6/1
  P/1 -> Gain1/1
  Square1/1 -> Sum/2
  Product3/1 -> Sum2/1
  Vectorized Clarke Transform/2(beta) -> Product3/1, Product2/1, Square1/1  "vbeta"
  Q/1 -> Gain/1
  "0 "/1 -> Vector Concatenate1/3
  Sum1/1 -> Product5/2
  Vectorized Inverse Clarke Transform/1(a) -> Vector Concatenate2/1
  Vectorized Inverse Clarke Transform/2(b) -> Vector Concatenate2/2
  Vectorized Clarke Transform/3(zero) -> Terminator6/1
  Product2/1 -> Sum1/2
  Vectorized Clarke Transform/1(alpha) -> Product4/1, Product1/1, Square/1  "valpha"
  Product6/1 -> Vector Concatenate1/2
  Product4/1 -> Sum2/2
  Vectorized Inverse Clarke Transform/3(c) -> Vector Concatenate2/3
  Product1/1 -> Sum1/1
  Vector Concatenate1/1 -> Vectorized Inverse Clarke Transform/1(alphabeta0)
  Square/1 -> Sum/1
  Product5/1 -> Vector Concatenate1/1
  Vectorized PQ meas/1(P) -> Terminator1/1  "P"
  Vectorized PQ meas/2(Q) -> Terminator2/1  "Q"
  Vector Concatenate2/1 -> Selector/1, Vectorized PQ meas/2(I)
  Vectorized Park Transform/1(d) -> Vector Concatenate3/1
  Vectorized Park Transform/2(q) -> Vector Concatenate3/2
  Vectorized Park Transform/3(0) -> Vector Concatenate3/3
  Vectorized Inverse Park Transform/1(a) -> Vector Concatenate4/1
  Vectorized Inverse Park Transform/2(b) -> Vector Concatenate4/2
  Vectorized Inverse Park Transform/3(c) -> Vector Concatenate4/3
  Vector Concatenate4/1 -> Vectorized Clarke Transform/1(abc), Vectorized PQ meas/1(V)
  Constant/1 -> Discrete-Time Integrator/1
  Discrete-Time Integrator/1 -> Vectorized Inverse Park Transform/2(theta), Vectorized Park Transform/2(theta)
  Vector Concatenate3/1 -> Subsystem/1(In1)
  Subsystem/1(Out1) -> Vectorized Inverse Park Transform/1(dq0)
  Transport Delay3/1 -> Mux/3
  meas/1 -> Transport Delay3/1, Transport Delay2/1, Mux/1
  Transport Delay2/1 -> Mux/2
  Gain/1 -> Product4/2, Product2/2
  Gain1/1 -> Product1/2, Product3/2
  Mux/1 -> Vectorized Park Transform/1(abc)  "vABC"
  Selector/1 -> I_1ph/1

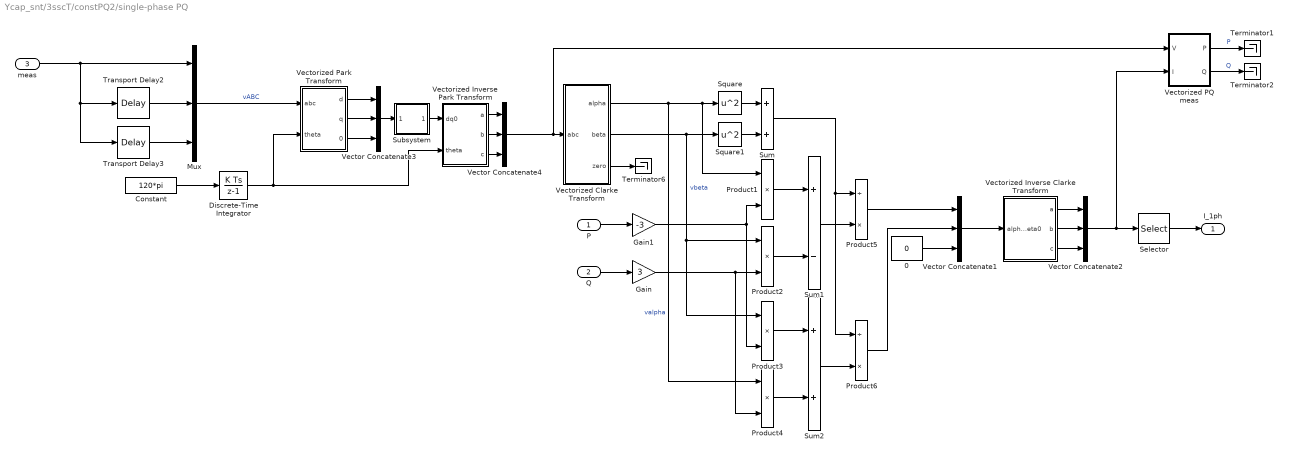
== system Ycap_snt/3sscT/constPQ2/single-phase PQ ==
  P : Inport
  Q : Inport  Port=2
  meas : Inport  Port=3
  "0 " : Constant  Value=0  VectorParams1D=off  SampleTime=Ts
  Constant : Constant  Value=120*pi  VectorParams1D=off  SampleTime=Ts
  Discrete-Time Integrator : DiscreteIntegrator  SampleTime=Ts  ICPrevOutput=DiscIntNeverNeededParam  ICPrevScaledInput=DiscIntNeverNeededParam
  Gain : Gain  Gain=3
  Gain1 : Gain  Gain=-3
  Mux : Mux  Inputs=3
  Product{1..4} (4 alike) : Product
  Product5 : Product  Inputs=/*
  Product6 : Product  Inputs=/*
  Selector : Selector  InputPortWidth=3  IndexOptions=Index vector (dialog)  Indices=1  OutputSizes=1
  Square : Math  Operator=square
  Square1 : Math  Operator=square
  Subsystem : Subsystem
  Sum : Sum
  Sum1 : Sum  Inputs=+-
  Sum2 : Sum
  Terminator1 : Terminator
  Terminator2 : Terminator
  Terminator6 : Terminator
  Transport Delay2 : TransportDelay  DelayTime=1/180
  Transport Delay3 : TransportDelay  DelayTime=2/180
  Vector Concatenate{1..4} (4 alike) : Concatenate  NumInputs=3  Mode=Multidimensional array
  Vectorized Clarke Transform : Subsystem  mask{no_meas=1}
      mask prompts: no_meas "Number of measurements"
  Vectorized PQ meas : Subsystem  DialogController=POWERSYS.PowerSysDialog
  Vectorized Park Transform : Subsystem  mask{no_meas=1}
      mask prompts: no_meas "Number of measurements"
  Vectorized Inverse Clarke Transform : Subsystem  mask{no_meas=1}
      mask prompts: no_meas "Number of Measurements"
      mask Display:
      | port_label('input', 1, '\alpha\beta0', 'texmode', 'on')
      | port_label('output',1,'a')
      | port_label('output',2,'b')
      | port_label('output',3,'c')
  Vectorized Inverse Park Transform : Subsystem  mask{no_meas=1}
      mask prompts: no_meas "Number of Measurements"
  I_1ph : Outport
  wires:
  Selector/1 -> I_1ph/1
  Mux/1 -> Vectorized Park Transform/1(abc)  "vABC"
  Gain1/1 -> Product3/2, Product1/2
  Gain/1 -> Product2/2, Product4/2
  Transport Delay2/1 -> Mux/2
  meas/1 -> Mux/1, Transport Delay2/1, Transport Delay3/1
  Transport Delay3/1 -> Mux/3
  Subsystem/1(Out1) -> Vectorized Inverse Park Transform/1(dq0)
  Vector Concatenate3/1 -> Subsystem/1(In1)
  Discrete-Time Integrator/1 -> Vectorized Park Transform/2(theta), Vectorized Inverse Park Transform/2(theta)
  Constant/1 -> Discrete-Time Integrator/1
  Vector Concatenate4/1 -> Vectorized PQ meas/1(V), Vectorized Clarke Transform/1(abc)
  Vectorized Inverse Park Transform/3(c) -> Vector Concatenate4/3
  Vectorized Inverse Park Transform/2(b) -> Vector Concatenate4/2
  Vectorized Inverse Park Transform/1(a) -> Vector Concatenate4/1
  Vectorized Park Transform/3(0) -> Vector Concatenate3/3
  Vectorized Park Transform/2(q) -> Vector Concatenate3/2
  Vectorized Park Transform/1(d) -> Vector Concatenate3/1
  Vector Concatenate2/1 -> Vectorized PQ meas/2(I), Selector/1
  Vectorized PQ meas/2(Q) -> Terminator2/1  "Q"
  Vectorized PQ meas/1(P) -> Terminator1/1  "P"
  Product5/1 -> Vector Concatenate1/1
  Square/1 -> Sum/1
  Vector Concatenate1/1 -> Vectorized Inverse Clarke Transform/1(alphabeta0)
  Product1/1 -> Sum1/1
  Vectorized Inverse Clarke Transform/3(c) -> Vector Concatenate2/3
  Product4/1 -> Sum2/2
  Product6/1 -> Vector Concatenate1/2
  Vectorized Clarke Transform/1(alpha) -> Square/1, Product1/1, Product4/1  "valpha"
  Product2/1 -> Sum1/2
  Vectorized Clarke Transform/3(zero) -> Terminator6/1
  Vectorized Inverse Clarke Transform/2(b) -> Vector Concatenate2/2
  Vectorized Inverse Clarke Transform/1(a) -> Vector Concatenate2/1
  Sum1/1 -> Product5/2
  "0 "/1 -> Vector Concatenate1/3
  Q/1 -> Gain/1
  Vectorized Clarke Transform/2(beta) -> Square1/1, Product2/1, Product3/1  "vbeta"
  Product3/1 -> Sum2/1
  Square1/1 -> Sum/2
  P/1 -> Gain1/1
  Sum/1 -> Product6/1, Product5/1
  Sum2/1 -> Product6/2

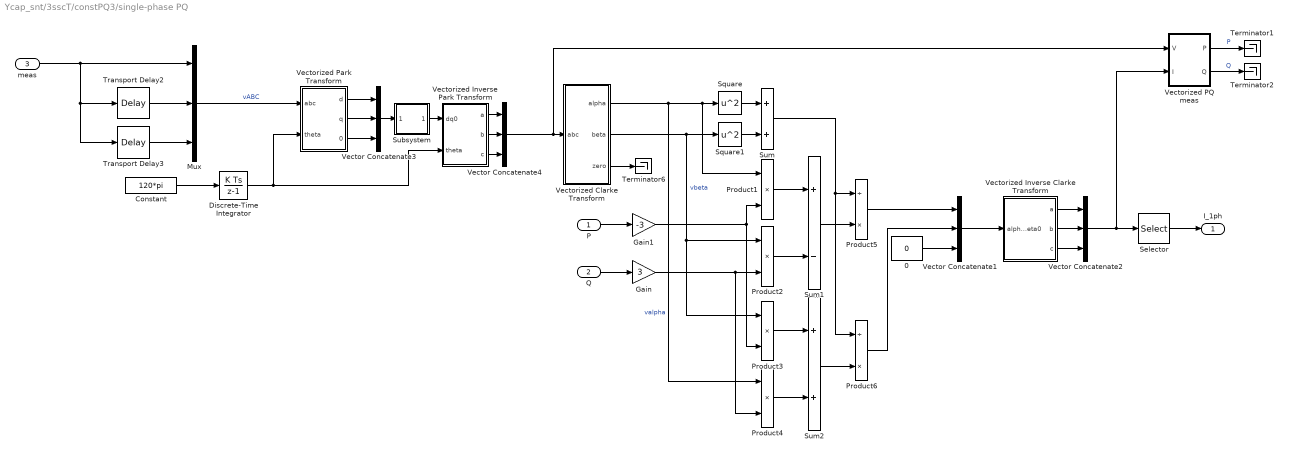
== system Ycap_snt/3sscT/constPQ3/single-phase PQ ==
  P : Inport
  Q : Inport  Port=2
  meas : Inport  Port=3
  "0 " : Constant  Value=0  VectorParams1D=off  SampleTime=Ts
  Constant : Constant  Value=120*pi  VectorParams1D=off  SampleTime=Ts
  Discrete-Time Integrator : DiscreteIntegrator  SampleTime=Ts  ICPrevOutput=DiscIntNeverNeededParam  ICPrevScaledInput=DiscIntNeverNeededParam
  Gain : Gain  Gain=3
  Gain1 : Gain  Gain=-3
  Mux : Mux  Inputs=3
  Product{1..4} (4 alike) : Product
  Product5 : Product  Inputs=/*
  Product6 : Product  Inputs=/*
  Selector : Selector  InputPortWidth=3  IndexOptions=Index vector (dialog)  Indices=1  OutputSizes=1
  Square : Math  Operator=square
  Square1 : Math  Operator=square
  Subsystem : Subsystem
  Sum : Sum
  Sum1 : Sum  Inputs=+-
  Sum2 : Sum
  Terminator1 : Terminator
  Terminator2 : Terminator
  Terminator6 : Terminator
  Transport Delay2 : TransportDelay  DelayTime=1/180
  Transport Delay3 : TransportDelay  DelayTime=2/180
  Vector Concatenate{1..4} (4 alike) : Concatenate  NumInputs=3  Mode=Multidimensional array
  Vectorized Clarke Transform : Subsystem  mask{no_meas=1}
      mask prompts: no_meas "Number of measurements"
  Vectorized PQ meas : Subsystem  DialogController=POWERSYS.PowerSysDialog
  Vectorized Park Transform : Subsystem  mask{no_meas=1}
      mask prompts: no_meas "Number of measurements"
  Vectorized Inverse Clarke Transform : Subsystem  mask{no_meas=1}
      mask prompts: no_meas "Number of Measurements"
      mask Display:
      | port_label('input', 1, '\alpha\beta0', 'texmode', 'on')
      | port_label('output',1,'a')
      | port_label('output',2,'b')
      | port_label('output',3,'c')
  Vectorized Inverse Park Transform : Subsystem  mask{no_meas=1}
      mask prompts: no_meas "Number of Measurements"
  I_1ph : Outport
  wires:
  Sum2/1 -> Product6/2
  Sum/1 -> Product5/1, Product6/1
  P/1 -> Gain1/1
  Square1/1 -> Sum/2
  Product3/1 -> Sum2/1
  Vectorized Clarke Transform/2(beta) -> Product3/1, Product2/1, Square1/1  "vbeta"
  Q/1 -> Gain/1
  "0 "/1 -> Vector Concatenate1/3
  Sum1/1 -> Product5/2
  Vectorized Inverse Clarke Transform/1(a) -> Vector Concatenate2/1
  Vectorized Inverse Clarke Transform/2(b) -> Vector Concatenate2/2
  Vectorized Clarke Transform/3(zero) -> Terminator6/1
  Product2/1 -> Sum1/2
  Vectorized Clarke Transform/1(alpha) -> Product4/1, Product1/1, Square/1  "valpha"
  Product6/1 -> Vector Concatenate1/2
  Product4/1 -> Sum2/2
  Vectorized Inverse Clarke Transform/3(c) -> Vector Concatenate2/3
  Product1/1 -> Sum1/1
  Vector Concatenate1/1 -> Vectorized Inverse Clarke Transform/1(alphabeta0)
  Square/1 -> Sum/1
  Product5/1 -> Vector Concatenate1/1
  Vectorized PQ meas/1(P) -> Terminator1/1  "P"
  Vectorized PQ meas/2(Q) -> Terminator2/1  "Q"
  Vector Concatenate2/1 -> Selector/1, Vectorized PQ meas/2(I)
  Vectorized Park Transform/1(d) -> Vector Concatenate3/1
  Vectorized Park Transform/2(q) -> Vector Concatenate3/2
  Vectorized Park Transform/3(0) -> Vector Concatenate3/3
  Vectorized Inverse Park Transform/1(a) -> Vector Concatenate4/1
  Vectorized Inverse Park Transform/2(b) -> Vector Concatenate4/2
  Vectorized Inverse Park Transform/3(c) -> Vector Concatenate4/3
  Vector Concatenate4/1 -> Vectorized Clarke Transform/1(abc), Vectorized PQ meas/1(V)
  Constant/1 -> Discrete-Time Integrator/1
  Discrete-Time Integrator/1 -> Vectorized Inverse Park Transform/2(theta), Vectorized Park Transform/2(theta)
  Vector Concatenate3/1 -> Subsystem/1(In1)
  Subsystem/1(Out1) -> Vectorized Inverse Park Transform/1(dq0)
  Transport Delay3/1 -> Mux/3
  meas/1 -> Transport Delay3/1, Transport Delay2/1, Mux/1
  Transport Delay2/1 -> Mux/2
  Gain/1 -> Product4/2, Product2/2
  Gain1/1 -> Product1/2, Product3/2
  Mux/1 -> Vectorized Park Transform/1(abc)  "vABC"
  Selector/1 -> I_1ph/1

== system Ycap_snt/1sscT/constPQ1/single-phase PQ/Subsystem ==
  In1 : Inport
  Discrete-Time Integrator : DiscreteIntegrator  gainval=1/Ts/20  InitialCondition=2000  SampleTime=-1  ICPrevOutput=DiscIntNeverNeededParam  ICPrevScaledInput=DiscIntNeverNeededParam
  Sum : Sum  Inputs=|+-
  Out1 : Outport
  wires:
  In1/1 -> Sum/1
  Sum/1 -> Discrete-Time Integrator/1
  Discrete-Time Integrator/1 -> Sum/2, Out1/1

== system Ycap_snt/1sscT/constPQ1/single-phase PQ/Vectorized Clarke Transform ==
  abc : Inport
  Constant1 : Constant  Value=-0.5*ones(1,no_meas)  VectorParams1D=off  SampleTime=Ts
  Constant{2..4,6} (4 alike) : Constant  Value=ones(1,no_meas)  VectorParams1D=off  SampleTime=Ts
  Constant5 : Constant  Value=-0.5*ones(1,no_meas)  VectorParams1D=off  SampleTime=Ts
  Constant7 : Constant  Value=zeros(1,no_meas)  VectorParams1D=off  SampleTime=Ts
  Constant8 : Constant  Value=sqrt(3)/2*ones(1,no_meas)  VectorParams1D=off  SampleTime=Ts
  Constant9 : Constant  Value=-sqrt(3)/2*ones(1,no_meas)  VectorParams1D=off  SampleTime=Ts
  Gain : Gain  Gain=sqrt(2/3)
  Gain1 : Gain  Gain=sqrt(2/3)
  Gain2 : Gain  Gain=sqrt(1/3)
  Product : Product
  Product1 : Product
  Product2 : Product
  Sum2 : Sum  Inputs=1  CollapseMode=Specified dimension  InputSameDT=on  SaturateOnIntegerOverflow=on  OutDataTypeStr=Inherit: Same as first input
  Sum3 : Sum  Inputs=1  CollapseMode=Specified dimension  InputSameDT=on  SaturateOnIntegerOverflow=on  OutDataTypeStr=Inherit: Same as first input
  Sum4 : Sum  Inputs=1  CollapseMode=Specified dimension  InputSameDT=on  SaturateOnIntegerOverflow=on  OutDataTypeStr=Inherit: Same as first input
  Vector Concatenate1 : Concatenate  NumInputs=3  Mode=Multidimensional array
  Vector Concatenate2 : Concatenate  NumInputs=3  Mode=Multidimensional array
  Vector Concatenate3 : Concatenate  NumInputs=3  Mode=Multidimensional array
  alpha : Outport  VectorParamsAs1DForOutWhenUnconnected=off
  beta : Outport  Port=2  VectorParamsAs1DForOutWhenUnconnected=off
  zero : Outport  Port=3  VectorParamsAs1DForOutWhenUnconnected=off
  wires:
  Gain/1 -> alpha/1
  Gain1/1 -> beta/1
  Gain2/1 -> zero/1
  Sum2/1 -> Gain/1
  Sum4/1 -> Gain2/1
  Sum3/1 -> Gain1/1
  Product2/1 -> Sum4/1
  Product1/1 -> Sum3/1
  Product/1 -> Sum2/1
  Vector Concatenate1/1 -> Product/2
  Vector Concatenate2/1 -> Product1/2
  Vector Concatenate3/1 -> Product2/2
  Constant3/1 -> Vector Concatenate3/3
  Constant2/1 -> Vector Concatenate3/2
  Constant4/1 -> Vector Concatenate3/1
  abc/1 -> Product/1, Product1/1, Product2/1
  Constant6/1 -> Vector Concatenate1/1
  Constant1/1 -> Vector Concatenate1/2
  Constant5/1 -> Vector Concatenate1/3
  Constant7/1 -> Vector Concatenate2/1
  Constant8/1 -> Vector Concatenate2/2
  Constant9/1 -> Vector Concatenate2/3
